simulink model "snowpack_melt"  (R2014a)
settings: Solver=ode45  StartTime=0.0  StopTime=10.0  RelTol=1e-3
undefined symbols (not defined in the file): As, Bs, Cs, DiscIntNeverNeededParam, Lf
settings Model: Creator=feisele  LastModifiedBy=feisele

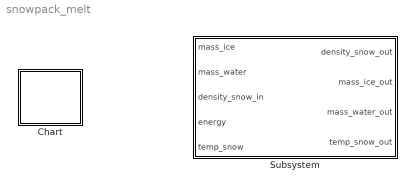
== system snowpack_melt ==
  Chart : Stateflow chart  TreatAsAtomicUnit=on
  Subsystem : Subsystem

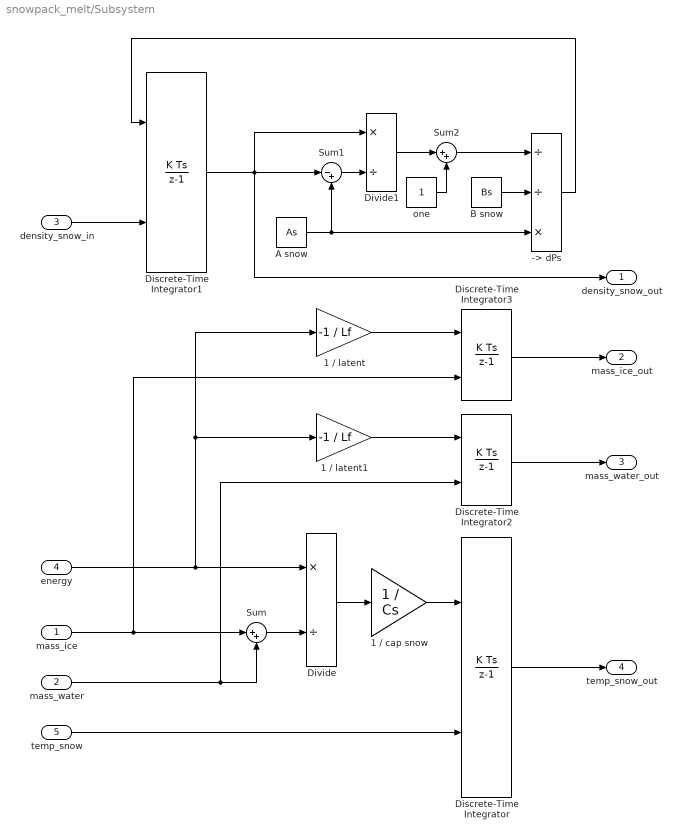
== system snowpack_melt/Subsystem ==
  mass_ice : Inport
  mass_water : Inport  Port=2
  density_snow_in : Inport  Port=3
  energy : Inport  Port=4
  temp_snow : Inport  Port=5
  -> dPs : Product  Inputs=//*
  1 / cap snow : Gain  Gain=1 / Cs
  1 / latent : Gain  Gain=-1 / Lf
  1 / latent1 : Gain  Gain=-1 / Lf
  A snow : Constant  Value=As
  B snow : Constant  Value=Bs
  Discrete-Time Integrator{,1..3} (4 alike) : DiscreteIntegrator  InitialConditionSource=external  SampleTime=-1  ICPrevOutput=DiscIntNeverNeededParam  ICPrevScaledInput=DiscIntNeverNeededParam
  Divide : Product  Inputs=*/
  Divide1 : Product  Inputs=*/
  Sum : Sum  Inputs=|++
  Sum1 : Sum  Inputs=|-+
  Sum2 : Sum  Inputs=|++
  one : Constant
  density_snow_out : Outport
  mass_ice_out : Outport  Port=2
  mass_water_out : Outport  Port=3
  temp_snow_out : Outport  Port=4
  wires:
  density_snow_in/1 -> Discrete-Time Integrator1/2
  Discrete-Time Integrator1/1 -> density_snow_out/1, Divide1/1, Sum1/1
  A snow/1 -> Sum1/2, -> dPs/3
  Divide1/1 -> Sum2/1
  one/1 -> Sum2/2
  Sum2/1 -> -> dPs/1
  Sum1/1 -> Divide1/2
  B snow/1 -> -> dPs/2
  -> dPs/1 -> Discrete-Time Integrator1/1
  Discrete-Time Integrator/1 -> temp_snow_out/1
  Divide/1 -> 1 / cap snow/1
  1 / cap snow/1 -> Discrete-Time Integrator/1
  energy/1 -> Divide/1, 1 / latent/1, 1 / latent1/1
  temp_snow/1 -> Discrete-Time Integrator/2
  mass_ice/1 -> Discrete-Time Integrator3/2, Sum/1
  Sum/1 -> Divide/2
  Discrete-Time Integrator3/1 -> mass_ice_out/1
  1 / latent/1 -> Discrete-Time Integrator3/1
  mass_water/1 -> Discrete-Time Integrator2/2, Sum/2
  1 / latent1/1 -> Discrete-Time Integrator2/1
  Discrete-Time Integrator2/1 -> mass_water_out/1

== stateflow chart snowpack_melt/Chart ==
